simulink model "Assignment_3_lqr"  (R2019b)
settings: Solver=VariableStepAuto  StartTime=0.0  StopTime=10.0  RelTol=1e-3
undefined symbols (not defined in the file): A, B, C, K, x0
settings Model: Creator=Vishrant  LastModifiedBy=Vishrant

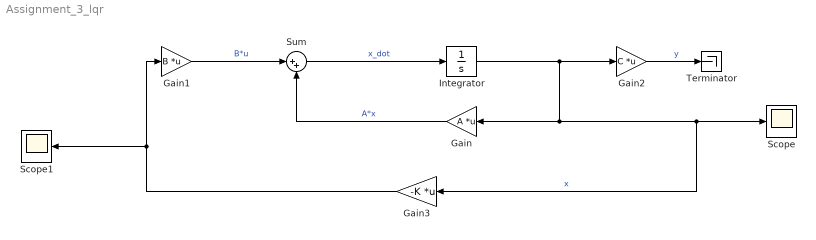
== system Assignment_3_lqr ==
  Gain : Gain  Gain=A  Multiplication=Matrix(K*u)
  Gain1 : Gain  Gain=B  Multiplication=Matrix(K*u)
  Gain2 : Gain  Gain=C  Multiplication=Matrix(K*u)
  Gain3 : Gain  Gain=-K  Multiplication=Matrix(K*u)
  Integrator : Integrator  InitialCondition=x0
  Scope : Scope
  Scope1 : Scope
  Sum : Sum  Inputs=|++
  Terminator : Terminator
  wires:
  Gain/1 -> Sum/2  "A*x"
  Integrator/1 -> Gain2/1, Gain/1, Scope/1, Gain3/1  "x"
  Sum/1 -> Integrator/1  "x_dot"
  Gain1/1 -> Sum/1  "B*u"
  Gain3/1 -> Gain1/1, Scope1/1
  Gain2/1 -> Terminator/1  "y"
